simulink model "deneme3"  (R2023b)
settings: Solver=VariableStepAuto  StartTime=0.0  StopTime=10000  RelTol=1e-3
libraries: shared6dof x1, robotcorelib x1, sim3dlib x1, uavsim3dlib x1
settings Model: Creator=SafakPC  LastModifiedBy=SafakPC

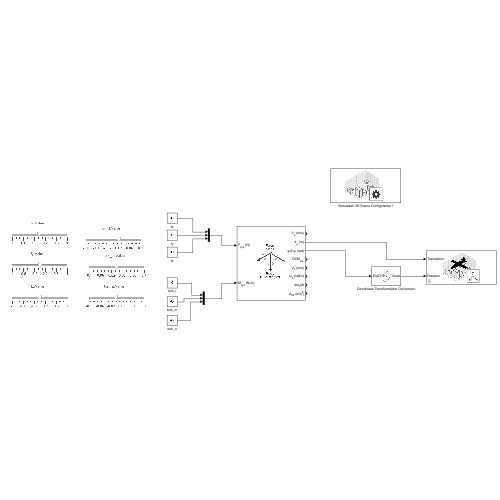
[thumbnail: Simulink's stored preview of the top-level diagram]
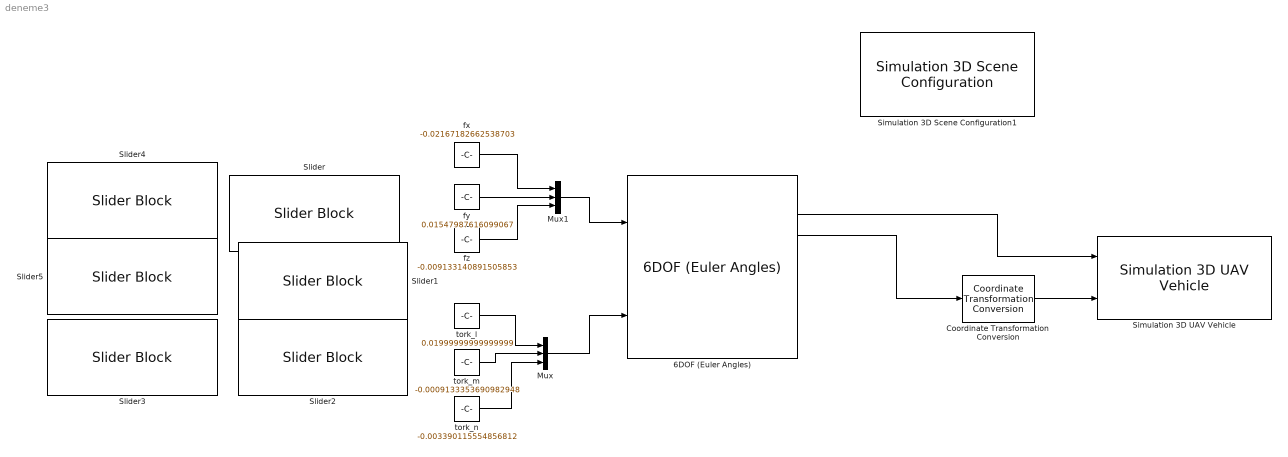
== system deneme3 ==
  6DOF (Euler Angles) : shared6dof/6DOF (Euler Angles)  units=Metric (MKS)  mtype=Fixed  rep=Euler Angles  xme_0=[0 0 0]  Vm_0=[0 0 0]  eul_0=[0 0 0]  pm_0=[0 0 0]  mass_0=1.0  mass_e=0.5  mass_f=2.0  inertia=eye(3)  inertia_e=eye(3)  inertia_f=2*eye(3)  k_quat=1.0  vre_flag=on  abi_flag=off  aMode=0  xme_statename=''  Vm_statename=''  eul_statename=''  quat_statename=''  pm_statename=''  mass_statename=''
  Coordinate Transformation Conversion : robotcorelib/Coordinate Transformation Conversion  InputRepresentation=Euler Angles  InputEulerSequence=ZYX  ShowTrVecInputPort=on  OutputRepresentation=Quaternion  OutputEulerSequence=ZYX  ShowTrVecOutputPort=on  SimulateUsing=Interpreted execution
      settings: LibrarySourceBlock=uavutilslib/Coordinate Transformation Conversion
  Mux : Mux  Inputs=3
  Mux1 : Mux  Inputs=3
  Simulation 3D Scene Configuration1 : sim3dlib/Simulation 3D Scene Configuration  Priority=0  ProjectFormat=Default Scenes  SceneDesc=US city block  ProjectName=C:\Program Files\MATLAB\R2023b\toolbox\shared\sim3d_projects\automotive_project_windows\UE\WindowsNoEditor\VehicleSimulation.exe  ScenePath=/Game/Maps/USCityBlock  EnableOpenDRIVE=off  vehTagList={'Custom';'Scene Origin';'SimulinkVehicle1'}  vehTag=SimulinkVehicle1  FreeCameraInitialTranslation=[0, 0, 0]  FreeCameraDefaultInitialTranslation=[-6, 0, 2]  FreeCameraInitialRotation=[0, 0, 0]  FreeCameraDefaultInitialRotation=[0, -15, 0]  OpVisEn=off  Ts=1/60  EnableWindow=on  EnableRemoteAccess=off  EnableWeather=off  SunAltitude=40.0  SunAzimuth=90  clouds=10  wind=1  fog=0  rain=0  EnableGeospatial=off  OriginHeight=200  OriginLatitude=40.744652  OriginLongitude=-73.988864  MapStyle=Aerial  AdditionalAssetIDs=[]  UseAdvancedSunSky=off  SolarTime=11  TimeZone=-5  Day=21  Month=9  Year=2022  UseDaylightSavingTime=on  DSTStartDay=10  DSTStartMonth=3  DSTEndDay=3  DSTEndMonth=11  DSTSwitchHour=2  sensorTag=MainCamera2  sensorId=2  sensorName=MainCamera2  mountLoc=Origin  offsetFlag=off  tmountOffset=[0, 0, 0]  rmountOffset=[0, 0, 0]  HorizontalResolution=1280  VerticalResolution=720  HorizontalFOV=60  mountPoint=[0 0 0]  mountOrientation=[0 0 0]  aMode=4  ID=2  GeoTrigger=Inactive
      settings: LibrarySourceBlock=uavsim3dlib/Simulation 3D Scene Configuration
  Simulation 3D UAV Vehicle : uavsim3dlib/Simulation 3D UAV Vehicle  Priority=-1  Mesh=Fixed wing  MeshPath=/MathWorksUAVContent/UAVs/HexaRotorUAV/HexaRotor.HexaRotor  Color=Yellow  ActorName=SimulinkVehicle1  UseGlobalFrame=off  InitialTranslation=[100 100 100]  InitialRotation=[0 0 0]  InitialTranslationGlobal=[0 0 0]  InitialGeoOrigin=[0 0 0]  InitialRotationGlobal=[0 0 0]  SampleTime=-1  ActorType=SimulinkVehicle  ID=1  aMode=4  ActorTag=SimulinkVehicle1
  Slider : SliderBlock  ScaleMin=-0.1  ScaleMax=0.1
  Slider1 : SliderBlock  ScaleMin=-0.1  ScaleMax=0.1
  Slider2 : SliderBlock  ScaleMin=-0.1  ScaleMax=0.1
  Slider3 : SliderBlock  ScaleMin=-1  ScaleMax=1
  Slider4 : SliderBlock  ScaleMin=-1  ScaleMax=1
  Slider5 : SliderBlock  ScaleMin=-1  ScaleMax=1
  fx : Constant  Value=-0.02167182662538703
  fy : Constant  Value=0.01547987616099067
  fz : Constant  Value=-0.009133140891505853
  tork_l : Constant  Value=0.01999999999999999
  tork_m : Constant  Value=-0.0009133353690982948
  tork_n : Constant  Value=-0.003390115554856812
  wires:
  fz/1 -> Mux1/3
  Mux/1 -> 6DOF (Euler Angles)/2
  fy/1 -> Mux1/2
  tork_l/1 -> Mux/1
  Mux1/1 -> 6DOF (Euler Angles)/1
  tork_m/1 -> Mux/2
  tork_n/1 -> Mux/3
  fx/1 -> Mux1/1
  6DOF (Euler Angles)/3 -> Coordinate Transformation Conversion/1
  6DOF (Euler Angles)/2 -> Simulation 3D UAV Vehicle/1
  Coordinate Transformation Conversion/1 -> Simulation 3D UAV Vehicle/2
